simulink model "PMSM_FUZZY_CTRL"  (R2020a)
settings: Solver=VariableStepAuto  StartTime=0.0  StopTime=10.0  RelTol=1e-3
settings Model: Creator=LENOVO  LastModifiedBy=LENOVO

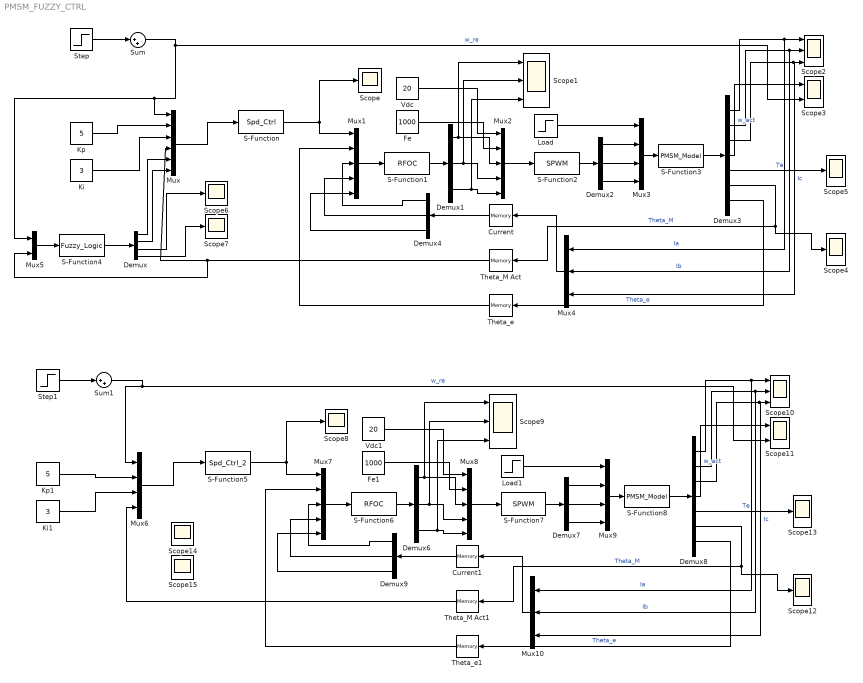
== system PMSM_FUZZY_CTRL ==
  Current : Memory
  Current1 : Memory
  Demux : Demux
  Demux{1..2,4,6..7,9} (6 alike) : Demux  Outputs=3
  Demux3 : Demux  Outputs=7
  Demux8 : Demux  Outputs=7
  Fe : Constant  Value=1000
  Fe1 : Constant  Value=1000
  Ki : Constant  Value=3
  Ki1 : Constant  Value=3
  Kp : Constant  Value=5
  Kp1 : Constant  Value=5
  Load : Step  Time=7  After=0.1  SampleTime=0
  Load1 : Step  Time=7  After=0.1  SampleTime=0
  Mux : Mux  Inputs=6
  Mux{1..2,7..8} (4 alike) : Mux  Inputs=5
  Mux10 : Mux  Inputs=3
  Mux3 : Mux
  Mux4 : Mux  Inputs=3
  Mux5 : Mux  Inputs=2
  Mux6 : Mux
  Mux9 : Mux
  S-Function : S-Function  FunctionName=Spd_Ctrl  SFunctionDeploymentMode=off  EnableBusSupport=off
  S-Function1 : S-Function  FunctionName=RFOC  SFunctionDeploymentMode=off  EnableBusSupport=off
  S-Function2 : S-Function  FunctionName=SPWM  SFunctionDeploymentMode=off  EnableBusSupport=off
  S-Function3 : S-Function  FunctionName=PMSM_Model  SFunctionDeploymentMode=off  EnableBusSupport=off
  S-Function4 : S-Function  FunctionName=Fuzzy_Logic  SFunctionDeploymentMode=off  EnableBusSupport=off
  S-Function5 : S-Function  FunctionName=Spd_Ctrl_2  SFunctionDeploymentMode=off  EnableBusSupport=off
  S-Function6 : S-Function  FunctionName=RFOC  SFunctionDeploymentMode=off  EnableBusSupport=off
  S-Function7 : S-Function  FunctionName=SPWM  SFunctionDeploymentMode=off  EnableBusSupport=off
  S-Function8 : S-Function  FunctionName=PMSM_Model  SFunctionDeploymentMode=off  EnableBusSupport=off
  Scope{,4..8,12..15} (10 alike) : Scope
  Scope{1..2,9..10} (4 alike) : Scope  NumInputPorts=3
  Scope11 : Scope  NumInputPorts=2
  Scope3 : Scope  NumInputPorts=2
  Step : Step  After=15  SampleTime=0
  Step1 : Step  After=15  SampleTime=0
  Sum : Sum  Inputs=|++
  Sum1 : Sum  Inputs=|++
  Theta_M Act : Memory
  Theta_M Act1 : Memory
  Theta_e : Memory
  Theta_e1 : Memory
  Vdc : Constant  Value=20
  Vdc1 : Constant  Value=20
  wires:
  Kp/1 -> Mux/2
  Ki/1 -> Mux/3
  Step/1 -> Sum/1
  Mux/1 -> S-Function/1
  Mux1/1 -> S-Function1/1
  S-Function1/1 -> Demux1/1
  Demux1/3 -> Scope1/3, Mux2/5
  Demux1/2 -> Mux2/4, Scope1/2
  Demux1/1 -> Scope1/1, Mux2/3
  Fe/1 -> Mux2/2
  Vdc/1 -> Mux2/1
  Mux2/1 -> S-Function2/1
  S-Function2/1 -> Demux2/1
  Demux2/3 -> Mux3/4
  Demux2/1 -> Mux3/2
  Demux2/2 -> Mux3/3
  Mux3/1 -> S-Function3/1
  Load/1 -> Mux3/1
  S-Function3/1 -> Demux3/1
  Demux3/1 -> Scope2/1, Mux4/1  "Ia"
  Demux3/2 -> Mux4/2, Scope2/2  "Ib"
  Demux3/3 -> Mux4/3, Scope2/3  "Ic"
  Demux3/4 -> Scope3/1  "w_act"
  Demux3/5 -> Scope5/1  "Te"
  Mux4/1 -> Current/1
  Demux3/6 -> Scope4/1, Theta_M Act/1  "Theta_M"
  Demux3/7 -> Theta_e/1  "Theta_e"
  Theta_e/1 -> Mux1/2
  Current/1 -> Demux4/1
  Demux4/1 -> Mux1/3
  Demux4/2 -> Mux1/4
  Demux4/3 -> Mux1/5
  Theta_M Act/1 -> Mux5/2, Mux/4
  Sum/1 -> Scope3/2, Mux/1, Mux5/1  "w_re"
  S-Function/1 -> Scope/1, Mux1/1
  Mux5/1 -> S-Function4/1
  S-Function4/1 -> Demux/1
  Demux/1 -> Mux/5
  Demux/2 -> Mux/6
  Demux/3 -> Scope6/1
  Demux/4 -> Scope7/1
  Sum1/1 -> Scope11/2, Mux6/1  "w_re"
  Theta_M Act1/1 -> Mux6/4
  Demux8/5 -> Scope13/1  "Te"
  Demux9/3 -> Mux7/5
  Fe1/1 -> Mux8/2
  Demux7/2 -> Mux9/3
  Demux8/6 -> Scope12/1, Theta_M Act1/1  "Theta_M"
  Demux8/1 -> Scope10/1, Mux10/1  "Ia"
  Demux8/7 -> Theta_e1/1  "Theta_e"
  Demux7/1 -> Mux9/2
  Mux9/1 -> S-Function8/1
  Theta_e1/1 -> Mux7/2
  Demux8/4 -> Scope11/1  "w_act"
  Demux8/3 -> Mux10/3, Scope10/3  "Ic"
  S-Function8/1 -> Demux8/1
  Demux6/2 -> Mux8/4, Scope9/2
  Vdc1/1 -> Mux8/1
  Demux9/2 -> Mux7/4
  S-Function5/1 -> Scope8/1, Mux7/1
  Demux7/3 -> Mux9/4
  Demux9/1 -> Mux7/3
  Demux6/1 -> Scope9/1, Mux8/3
  Mux7/1 -> S-Function6/1
  Step1/1 -> Sum1/1
  Load1/1 -> Mux9/1
  Demux6/3 -> Scope9/3, Mux8/5
  Mux6/1 -> S-Function5/1
  Ki1/1 -> Mux6/3
  S-Function7/1 -> Demux7/1
  Mux10/1 -> Current1/1
  Kp1/1 -> Mux6/2
  Mux8/1 -> S-Function7/1
  Current1/1 -> Demux9/1
  S-Function6/1 -> Demux6/1
  Demux8/2 -> Mux10/2, Scope10/2  "Ib"
